simulink model "CD_P6"  (R2020a)
settings: Solver=VariableStepAuto  StartTime=0.0  StopTime=1  RelTol=1e-3
settings Model: Creator=Usuario  LastModifiedBy=Usuario

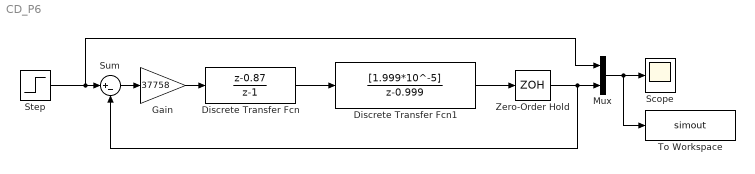
== system CD_P6 ==
  Discrete Transfer Fcn : DiscreteTransferFcn  Numerator=[1 -0.87]  Denominator=[1 -1]
  Discrete Transfer Fcn1 : DiscreteTransferFcn  Numerator=[1.999*10^-5]  Denominator=[1 -0.999]
  Gain : Gain  Gain=37758
  Mux : Mux  Inputs=2
  Scope : Scope
  Step : Step  Time=0  SampleTime=0
  Sum : Sum  Inputs=|+-
  To Workspace : ToWorkspace  VariableName=simout  SaveFormat=Timeseries  SampleTime=-1
  Zero-Order Hold : ZeroOrderHold  SampleTime=0.02
  wires:
  Gain/1 -> Discrete Transfer Fcn/1
  Step/1 -> Mux/1, Sum/1
  Sum/1 -> Gain/1
  Zero-Order Hold/1 -> Sum/2, Mux/2
  Discrete Transfer Fcn1/1 -> Zero-Order Hold/1
  Discrete Transfer Fcn/1 -> Discrete Transfer Fcn1/1
  Mux/1 -> To Workspace/1, Scope/1
